simulink model "SG_model"  (R2024b)
settings: Solver=VariableStepAuto  StartTime=0  StopTime=20  RelTol=1e-3
values from neighbouring files (symbols this model uses):
  Eff = @(x) Eff_p1*x.^9 + Eff_p2*x.^8 + Eff_p3*x.^7 + Eff_p4*x.^6 + Eff_p5*x.^5 + Eff_p6*x.^4 + Eff_p7*x.^3 + Eff_p8*x.^2 + Eff_p9*x + Eff_p10    [SG01_Flight_Dynamics.m]    (also in SG01_Flight_Dynamics_original.m = fit(Js, Effs, 'poly9'))
  initial_P = 0    [OpPointTest_main.m]    (also in SG_model_trim.m = op.states(4).x; trim_op_fixed_v.mat)
  initial_Pitch = -3.558    [OpPointTest_main.m]    (also in SG_model_trim.m = op.states(7).x; trim_op_fixed_v.mat = 0)
  initial_Q = 0    [OpPointTest_main.m]    (also in SG_model_trim.m = op.states(5).x; trim_op_fixed_v.mat)
  initial_R = 0    [OpPointTest_main.m]    (also in SG_model_trim.m = op.states(6).x; trim_op_fixed_v.mat)
  initial_ROLL = 0    [OpPointTest_main.m]    (also in SG_model_trim.m = op.states(8).x; trim_op_fixed_v.mat)
  initial_uspeed = 10.26    [OpPointTest_main.m]    (also in SG_model_trim.m = op.states(1).x; linear_model.mat = 10.285; trim_op_fixed_v.mat = 10.285)
  initial_vspeed = 0    [OpPointTest_main.m]    (also in SG_model_trim.m = op.states(2).x; trim_op_fixed_v.mat)
  initial_wspeed = -0.6383    [OpPointTest_main.m]    (also in SG_model_trim.m = op.states(3).x; trim_op_fixed_v.mat = 0)
  initial_YAW = 0    [OpPointTest_main.m]    (also in SG_model_trim.m = op.states(9).x; trim_op_fixed_v.mat)
  initial_Z = 100    [OpPointTest_main.m]    (also in SG_model_trim.m = op.states(10).x; trim_op_fixed_v.mat = -50)
settings Model: Creator=ricar  LastModifiedBy=ricar
settings DataIOCC: SaveFormat=StructureWithTime
settings OptimizationCC: BlockReduction=off  OptimizeBlockIOStorage=off  BufferReuse=off
settings DebuggingCC: AlgebraicLoopMsg=none

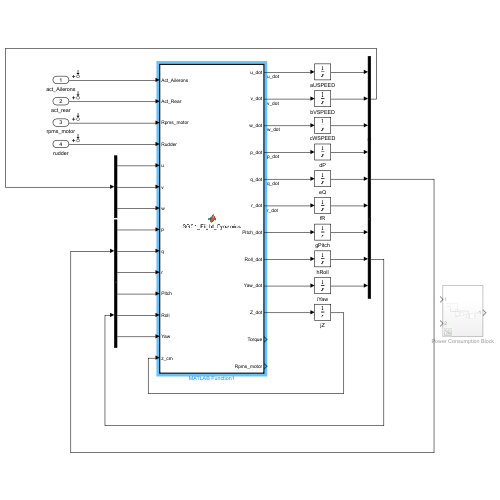
[thumbnail: Simulink's stored preview of the top-level diagram]
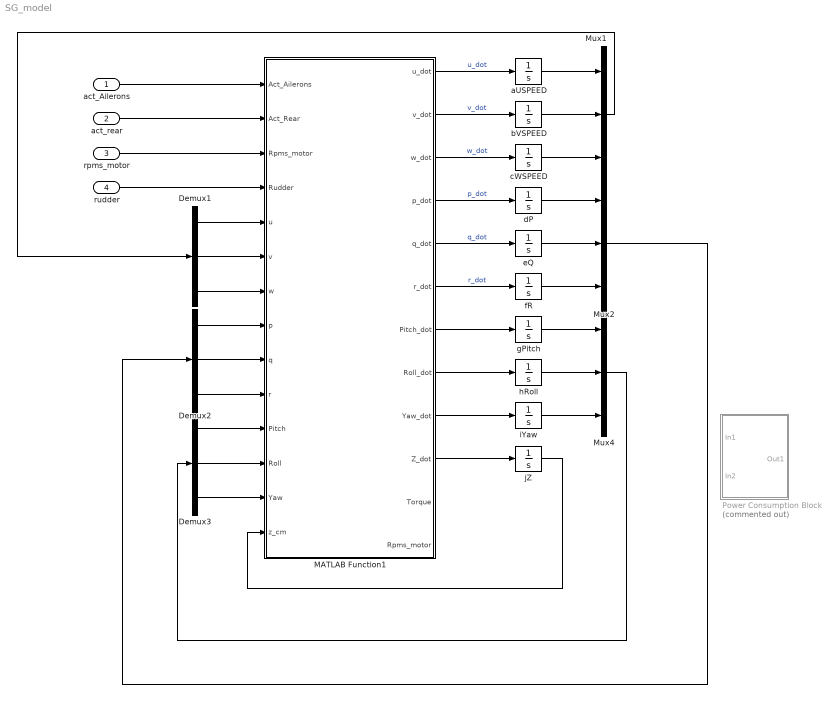
== system SG_model ==
  act_Ailerons : Inport
  act_rear : Inport  Port=2
  rpms_motor : Inport  Port=3
  rudder : Inport  Port=4
  Demux1 : Demux  Outputs=3
  Demux2 : Demux  Outputs=3
  Demux3 : Demux  Outputs=3
  MATLAB Function1 : MATLAB Function  TreatAsAtomicUnit=on
  Mux1 : Mux  Inputs=3
  Mux2 : Mux  Inputs=3
  Mux4 : Mux  Inputs=3
  Power Consumption Block : Subsystem  Commented=on
  aUSPEED : Integrator  InitialCondition=initial_uspeed
  bVSPEED : Integrator  InitialCondition=initial_vspeed
  cWSPEED : Integrator  InitialCondition=initial_wspeed
  dP : Integrator  InitialCondition=initial_P
  eQ : Integrator  InitialCondition=initial_Q
  fR : Integrator  InitialCondition=initial_R
  gPitch : Integrator  InitialCondition=initial_Pitch
  hRoll : Integrator  InitialCondition=initial_ROLL
  iYaw : Integrator  InitialCondition=initial_YAW
  jZ : Integrator  InitialCondition=initial_Z
  wires:
  jZ/1 -> MATLAB Function1/14(z_cm)
  iYaw/1 -> Mux4/3
  MATLAB Function1/4(p_dot) -> dP/1  "p_dot"
  MATLAB Function1/6(r_dot) -> fR/1  "r_dot"
  act_Ailerons/1 -> MATLAB Function1/1(Act_Ailerons)
  MATLAB Function1/2(v_dot) -> bVSPEED/1  "v_dot"
  MATLAB Function1/8(Roll_dot) -> hRoll/1
  act_rear/1 -> MATLAB Function1/2(Act_Rear)
  Mux4/1 -> Demux3/1
  dP/1 -> Mux2/1
  Mux2/1 -> Demux2/1
  MATLAB Function1/9(Yaw_dot) -> iYaw/1
  aUSPEED/1 -> Mux1/1
  Demux3/2 -> MATLAB Function1/12(Roll)
  MATLAB Function1/3(w_dot) -> cWSPEED/1  "w_dot"
  Demux2/3 -> MATLAB Function1/10(r)
  Demux3/1 -> MATLAB Function1/11(Pitch)
  MATLAB Function1/7(Pitch_dot) -> gPitch/1
  gPitch/1 -> Mux4/1
  eQ/1 -> Mux2/2
  Mux1/1 -> Demux1/1
  Demux1/3 -> MATLAB Function1/7(w)
  MATLAB Function1/5(q_dot) -> eQ/1  "q_dot"
  rudder/1 -> MATLAB Function1/4(Rudder)
  Demux1/1 -> MATLAB Function1/5(u)
  hRoll/1 -> Mux4/2
  cWSPEED/1 -> Mux1/3
  MATLAB Function1/1(u_dot) -> aUSPEED/1  "u_dot"
  Demux2/2 -> MATLAB Function1/9(q)
  Demux2/1 -> MATLAB Function1/8(p)
  Demux1/2 -> MATLAB Function1/6(v)
  rpms_motor/1 -> MATLAB Function1/3("Rpms_motor ")
  fR/1 -> Mux2/3
  Demux3/3 -> MATLAB Function1/13(Yaw)
  MATLAB Function1/10(Z_dot) -> jZ/1
  bVSPEED/1 -> Mux1/2

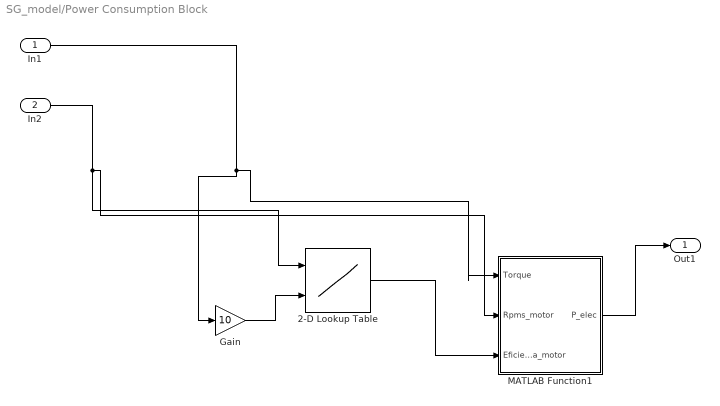
== system SG_model/Power Consumption Block ==
  In1 : Inport
  In2 : Inport  Port=2
  2-D Lookup Table : Lookup_n-D  BreakpointsForDimension1=[1:6000]  BreakpointsForDimension2=[1:140]  Table=Eff  InternalRulePriority=Speed  RndMeth=Simplest
      settings: InputPortMap=u0,u1
  Gain : Gain  Gain=10
  MATLAB Function1 : MATLAB Function  TreatAsAtomicUnit=on
  Out1 : Outport
  wires:
  In2/1 -> 2-D Lookup Table/1, MATLAB Function1/2(Rpms_motor)
  MATLAB Function1/1(P_elec) -> Out1/1
  In1/1 -> Gain/1, MATLAB Function1/1(Torque)
  Gain/1 -> 2-D Lookup Table/2
  2-D Lookup Table/1 -> MATLAB Function1/3(Eficiencia_motor)

== matlab function SG_model/MATLAB Function1 ==
  data: Act_Ailerons input; Act_Rear input; Rpms_motor input; Rudder input; u input; u_dot output; v input; w input; p input; q input; r input; Pitch input; Roll input; Yaw input; z_cm input; v_dot output; w_dot output; p_dot output; q_dot output; r_dot output; Pitch_dot output; Roll_dot output; Yaw_dot output; Z_dot output; Torque output; Rpms_motor output
function [u_dot,v_dot,w_dot,p_dot,q_dot,r_dot,Pitch_dot,Roll_dot,Yaw_dot,Z_dot,Torque,Rpms_motor] = SG01_Flight_Dynamics(Act_Ailerons,Act_Rear,Rpms_motor, Rudder,u,v,w,p,q,r,Pitch,Roll,Yaw,z_cm)

% Modelo Dinâmico do SG01, recebendo o estado do sistema ele retorna as
% derivadas das velocidades da "embarcação"

%%% CONSTANTES %%%

struts = 1;
wponto = 0;

g = 9.81; % Gravidade (m/s^2)
rho= 1026.00; % Densidade água salgada (kg/m^3)
mu= 1.14E-3; % Coef. viscosidade dinâmica água salgada (Pa*s)
m = 1500; % Massa da "embarcação" (Kg)
Ixx = 547.683;
Iyy = 3997.287; % Momentos de Inércia
Izz = 3782.999;
Ixz = -421.58174; % Produto de Inércia relevante
b = 2.400; % Span da Asa
c = 0.30988; % Corda média da Asa
S = 0.68757769; % Área da Asa
S_t = 0.20158673; % Área Elevator

if struts == 1 % struts estendidas, distancia submersa de strut
    z_struts = 1360 - z_cm/10; % estimativa muito rough
else
    z_struts = 0; % struts não estendidas INCLUIR AQUI TAMBÉM DIFERENTES DERIVADAS NO FUTURO
end


%%% DISTÂNCIAS %%% Esta secção deixou de ser necessária, acredito eu
x_cg_asas = 0.771; %centroide assumindo asa de tras semi eliptica e frente eliptica num referencial com origem a 20cm do leading edge da asa apontado para a cauda
X_CG_ASASRUDDERSTRUTS = (x_cg_asas*(S_t+S)-100*z_struts*2.825)/(S_t+S+100*z_struts); %X do CG das asa + rudder + struts no referencial com origem no meio da asa da frente CUIDADO COM O Z_STRUTS, que esta em mm
Z_CG_ASASRUDDERSTRUTS = (3*0.5*z_struts*100*z_struts)/(S_t+S+100*z_struts);
dist_CGSG_CGASAS_X = 3.715+X_CG_ASASRUDDERSTRUTS-3.964;
dist_CGSG_CGASAS_Y = 0; %idealmente
dist_CGSG_CGASAS_Z = z_struts + 1;

%%% Derivadas de estabilidade e controlo %%%
V = 10.28;
u0 = cos(deg2rad(-3.558))*V;
w0 = sin(deg2rad(-3.558))*V;
deltau = u - u0;
deltaw = w - w0;
deltaAct_Rear = Act_Rear - 4;
teta0 = -3.558;
Cw0 = (m*g*cos(teta0))/(0.5*rho*(u0^2)*S);
Cd1 = 0.015;

CXu = -0.02440;
CZu = -0.00701;
CMu = 0.08341;
CXa = 0.22694;
CLa = 5.93757;
CMa = -9.37193;
CXwponto = 0;
CLwponto = 0; % Não tenho como saber ainda
CMwponto = 0;
CXq = -0.31325;
CLq = 42.62028;
CMq = -319.07598;
CYb = -0.10815;
Clb = 0.11373;
CNb = 0.15492;
CYp = 0.18263;
Clp = -0.72524;
CNp = -0.33702;
CYr = 0.32068;
Clr = -0.22191;
CNr = -0.45556;
CXd_a = -0.00673;
CYd_a = 0.02042;
CZd_a = -0.26237;
Cld_a = 0.20542;
CMd_a = 0.06255;
CNd_a = -0.01074;
CXd_t = -0.01195;
CYd_t = 0; % meti a 0 porque não faz sentido
CZd_t = -1.20579;
Cld_t = 0;
CMd_t = -13.51024;
CNd_t = 0;
CXd_r = -0.01692;
CYd_r = 0.08540;
CZd_r = -0.35782;
Cld_r = -0.19211;
CMd_r = 0.13566;
CNd_r = -0.12412;

%%% DERIVADAS DIMENSIONAIS DE ESTABILIDADE %%

beta = asin(min(u/V,1));
alpha = atan(w/V);

Xu = rho*u0*S*sin(teta0)*Cw0 + 0.5*rho*S*u0*CXu;
Zu = -rho*u0*S*cos(teta0)*Cw0 + 0.5*rho*S*u0*CZu;
Mu = 0.5*rho*S*u0*c*CMu;
du = [Xu ; Zu ; Mu];

Xw = 0.5*rho*S*u0*CXa;
CZa = -(CLa + Cd1);
Zw = 0.5*rho*S*u0*CZa;
Mw = 0.5*rho*S*u0*CMa;
dw = [Xw ; Zw ; Mw];

Xwponto = 0.25*rho*S*c*CXwponto;
CZwponto = -CLwponto;
Zwponto = 0.25*rho*S*c*CZwponto;
Mwponto = 0.25*rho*S*c*c*CMwponto;
dwponto = [Xwponto ; Zwponto ; Mwponto];

Xq = 0.25*rho*S*u0*c*CXq;
CZq = -CLq;
Zq = 0.25*rho*S*u0*c*CZq;
Mq = 0.25*rho*S*u0*c*c*CMq;
dq = [Xq ; Zq ; Mq];

Yv = 0.25*rho*S*u0*CYb;
Lv = 0.5*rho*S*u0*beta*Clb;
Nv = 0.5*rho*S*u0*beta*CNb;
dv = [Yv ; Lv ; Nv];

Yp = 0.25*rho*u0*S*beta*CYp;
Lp = 0.25*rho*u0*S*beta*beta*Clp;
Np = 0.25*rho*u0*S*beta*beta*CNp;
dp = [Yp ; Lp ; Np];

Yr = 0.25*rho*S*u0*beta*CYr;
Lr = 0.25*rho*S*u0*beta*beta*Clr;
Nr = 0.25*rho*S*u0*beta*beta*CNr;
dr = [Yr ; Lr ; Nr];

%%% DERIVADAS DIMENSIONAIS CONTRLOLO EM RADIANOS%

Act_Ailerons = deg2rad(Act_Ailerons);
Act_Rear = deg2rad(Act_Rear);
Rudder = deg2rad(Rudder);

Xd_a = 0.5*rho*u0*u0*S*CXd_a;
Yd_a = 0.5*rho*u0*u0*S*CYd_a;
Zd_a = 0.5*rho*u0*u0*S*CZd_a;
Ld_a = 0.5*rho*u0*u0*S*beta*Cld_a;
Md_a = 0.5*rho*u0*u0*S*c*CMd_a;
Nd_a = 0.5*rho*u0*u0*S*beta*CNd_a;

Xd_t = 0.5*rho*u0*u0*S*CXd_t;
Yd_t = 0.5*rho*u0*u0*S*CYd_t;
Zd_t = 0.5*rho*u0*u0*S*CZd_t;
Ld_t = 0.5*rho*u0*u0*S*beta*Cld_t;
Md_t = 0.5*rho*u0*u0*S*c*CMd_t;
Nd_t = 0.5*rho*u0*u0*S*beta*CNd_t;

Xd_r = 0.5*rho*u0*u0*S*CXd_r;
Yd_r = 0.5*rho*u0*u0*S*CYd_r;
Zd_r = 0.5*rho*u0*u0*S*CZd_r;
Ld_r = 0.5*rho*u0*u0*S*beta*Cld_r;
Md_r = 0.5*rho*u0*u0*S*c*CMd_r;
Nd_r = 0.5*rho*u0*u0*S*beta*CNd_r;

%%% ALGURES CONDIÇÃO DE VENTILAÇÃO %%%

%%% THRUST %%%

Rpms_propeller = Rpms_motor/3;
diam = 0.335;

% Coefficients for KT 
KT_p1 = -39.575;
KT_p2 = 296.698;
KT_p3 = -977.420;
KT_p4 = 1855.793;
KT_p5 = -2236.302;
KT_p6 = 1772.128;
KT_p7 = -922.459;
KT_p8 = 303.597;
KT_p9 = -57.450;
KT_p10 = 5.070;

% KT function 
KT = @(x) KT_p1*x.^9 + KT_p2*x.^8 + KT_p3*x.^7 + KT_p4*x.^6 + KT_p5*x.^5 + KT_p6*x.^4 + KT_p7*x.^3 + KT_p8*x.^2 + KT_p9*x + KT_p10;

 
% Coefficients for kq 
Kq_p1 = 2.787;
Kq_p2 = -23.468;
Kq_p3 = 85.726;
Kq_p4 = -178.762;
Kq_p5 = 234.931;
Kq_p6 = -202.035;
Kq_p7 = 113.776;
Kq_p8 = -40.505;
Kq_p9 = 8.257;
Kq_p10 = -0.689;

% Kq function 
Kq = @(x) Kq_p1*x.^9 + Kq_p2*x.^8 + Kq_p3*x.^7 + Kq_p4*x.^6 + Kq_p5*x.^5 + Kq_p6*x.^4 + Kq_p7*x.^3 + Kq_p8*x.^2 + Kq_p9*x + Kq_p10;

 
Eff_p1 = -8627.603;
Eff_p2 = 61047.137;
Eff_p3 = -190004.847;
Eff_p4 = 341275.626;
Eff_p5 = -389694.487;
Eff_p6 = 293275.528;
Eff_p7 = -145425.793;
Eff_p8 = 45806.430;
Eff_p9 = -8313.959;
Eff_p10 = 662.694;
% Eff function 
Eff = @(x) Eff_p1*x.^9 + Eff_p2*x.^8 + Eff_p3*x.^7 + Eff_p4*x.^6 + Eff_p5*x.^5 + Eff_p6*x.^4 + Eff_p7*x.^3 + Eff_p8*x.^2 + Eff_p9*x + Eff_p10;

js = 60*V/(Rpms_propeller*diam);

kq = Kq(js);
kt = KT(js);
eff = Eff(js);

T = rho*(Rpms_propeller/60)^2*diam^4*kt;
P_propeller = T*V/eff;

%Calculate Power usage
P_mec=P_propeller/0.8;
Torque=P_mec/(Rpms_motor*2*pi/60);

%%% SOMATÓRIO %%%

X = du(1)*deltau + dw(1)*deltaw + dwponto(1)*wponto + dq(1)*q + Xd_a*Act_Ailerons + Xd_t*deltaAct_Rear + Xd_r*Rudder;
Y = dv(1)*v + dp(1)*p + dr(1)*r + Yd_a*Act_Ailerons + Yd_t*Act_Rear + Yd_r*Rudder;
Z = du(2)*deltau + dw(2)*deltaw + dwponto(2)*wponto + dq(2)*q + Zd_a*Act_Ailerons + Zd_t*deltaAct_Rear + Zd_r*Rudder;
L = dv(2)*v + dp(2)*p + dr(2)*r + Ld_a*Act_Ailerons + Ld_t*Act_Rear + Ld_r*Rudder;
M = du(3)*deltau + dw(3)*deltaw + dwponto(3)*wponto + dq(3)*q + Md_a*Act_Ailerons + Md_t*deltaAct_Rear + Md_r*Rudder;
N = dv(3)*v + dp(3)*p + dr(3)*r + Nd_a*Act_Ailerons + Nd_t*Act_Rear + Nd_r*Rudder;

%d = [dist_CGSG_CGASAS_X ; dist_CGSG_CGASAS_Y ; dist_CGSG_CGASAS_Z];
F = [X + T ; Y ; Z];
%M_1 = cross(d,F); não é necessário porque forças já estão no CG

M_2 = [L ; M ; N];

M_T = [0 ; 2.6 * T; 0]; % Momento só do Thrust, confia
Tau = M_2 + M_T; % Momentos livres + Momentos das Forças no CG do SG


%%% DERIVADAS %%%

R = [cosd(Pitch)*cosd(Yaw) cosd(Pitch)*sind(Yaw) -sind(Pitch);
    sind(Roll)*sind(Pitch)*cosd(Yaw)-cosd(Roll)*sind(Yaw) sind(Roll)*sind(Pitch)*sind(Yaw)+cosd(Roll)*cosd(Yaw) sind(Roll)*cosd(Pitch);
    cosd(Roll)*sind(Pitch)*cosd(Yaw)+sind(Roll)*sind(Yaw) cosd(Roll)*sind(Pitch)*sind(Yaw)-sind(Roll)*cosd(Yaw) cosd(Roll)*cosd(Pitch)]; % MATRIZ DE TRANSFERÊNCIA DE REFERENCIAL

%Balance of forces
p = p*pi/180;
q = q*pi/180;
r = r*pi/180;
ww = [p;q;r];

%W_inertial = m*g*[0;0;1];
W_inertial = 0;

uvw_dot = (F + R*W_inertial)/m - cross(ww, [u;v;w]);
VI_dot = R'*[u;v;w];

%Inertial angular velocities
Q = [1 sind(Roll)*tand(Pitch) cosd(Roll)*tand(Pitch);
     0 cosd(Roll) -sind(Roll);
     0 sind(Roll)/cosd(Pitch) cosd(Roll)/cosd(Pitch)];
eul = Q*ww;
Roll_dot = eul(1);
Pitch_dot = eul(2);
Yaw_dot = eul(3);

%Balance of moments

J = [Ixx 0 Ixz;
     0   Iyy 0;
     Ixz 0 Izz];
invJ = [-Izz/(Ixz^2 - Ixx*Izz),     0,  Ixz/(Ixz^2 - Ixx*Izz);
            0,                  1/Iyy,                      0;
       Ixz/(Ixz^2 - Ixx*Izz),     0,  -Ixx/(Ixz^2 - Ixx*Izz)];

wdot = invJ*(Tau - cross(ww,J*ww));

p_dot = wdot(1)*180/pi;
q_dot = wdot(2)*180/pi;
r_dot = wdot(3)*180/pi;

u_dot = uvw_dot(1);
v_dot = uvw_dot(2);
w_dot = uvw_dot(3);

Z_dot = VI_dot(3);
end

== matlab function SG_model/Power Consumption Block/MATLAB Function1 ==
  data: Torque input; P_elec output; Rpms_motor input; Eficiencia_motor input
function P_elec = fcn(Torque,Rpms_motor,Eficiencia_motor)
P_mec = Torque*Rpms_motor*2*pi/60;
P_elec = P_mec/Eficiencia_motor;
